simulink model "complementaryVsKalmanAndroidAHRS"  (R2019b)
settings: Solver=FixedStepAuto  StartTime=0.0  StopTime=40  RelTol=1e-3
InitFcn:
  | Ts=0.004
undefined symbols (not defined in the file): DiscIntNeverNeededParam
libraries: androiduilib x13, simulink_extras x11, dspstat3 x3, androidsensorlib x3
PreSaveFcn:
  | set_param(gcs, 'Location',[35 56 895 605])
settings Model: SimulationMode=external  ExtModeTrigDuration=100  Creator=The MathWorks, Inc.  LastModifiedBy=Alireza
settings DataIOCC: LimitDataPoints=on  SaveFormat=Array  ReturnWorkspaceOutputs=off
settings OptimizationCC: LifeSpan=1  MaxStackSize=64
settings DebuggingCC: UnderspecifiedInitializationDetection=Classic  MergeDetectMultiDrivingBlocksExec=none  ParameterPrecisionLossMsg=none  AllowSymbolicDim=off  SFUnexpectedBacktrackingDiag=warning  SFNoUnconditionalDefaultTransitionDiag=warning  SFExecutionAtInitializationDiag=none  ArithmeticOperatorsInVariantConditions=warning
settings HardwareCC: ProdBitPerPointer=32  ProdBitPerSizeT=32  ProdBitPerPtrDiffT=32  ProdLargestAtomicInteger=Long  ProdLargestAtomicFloat=Double  ProdWordSize=32  ProdHWDeviceType=ARM Compatible->ARM Cortex  TargetLargestAtomicInteger=Long  TargetLargestAtomicFloat=Double  TargetEndianess=LittleEndian  TargetHWDeviceType=ARM Compatible->ARM Cortex
settings ModelReferenceCC: PropagateSignalLabelsOutOfModel=off
settings SFSimCC: SimUseLocalCustomCode=off  CustomCodeUndefinedFunction=UseInterfaceOnly
settings RTWCC: SystemTargetFile=ert.tlc  HardwareBoard=Android Device  TLCOptions="-aInlineSetEventsForThisBaseRateFcn=TLC_FALSE -aSuppressMultiTaskScheduler=TLC_FALSE  -aRateBasedStepFcn=0"  TemplateMakefile=ert_default_tmf  GenerateReport=on  RTWVerbose=off  RTWUseLocalCustomCode=off  Toolchain=Android SDK/NDK Tools  LaunchReport=on
settings CodeAppCC: ForceParamTrailComments=on  OperatorAnnotations=on  MangleLength=10  StateflowObjectComments=on  MATLABSourceComments=on
settings ERTTargetCC: MultiwordLength=2048  ERTCustomFileBanners=off  SupportContinuousTime=on  SupportNonInlinedSFcns=on  RemoveResetFunc=off  SupportVariableSizeSignals=on  ModelStepFunctionPrototypeControlCompliant=off
settings ConfigComp: CovMetricSettings=dw  CovHtmlReporting=on  CovSaveCumulativeToWorkspaceVar=on  CovSaveSingleToWorkspaceVar=on  CovExternalEMLEnable=off  CovSFcnEnable=off

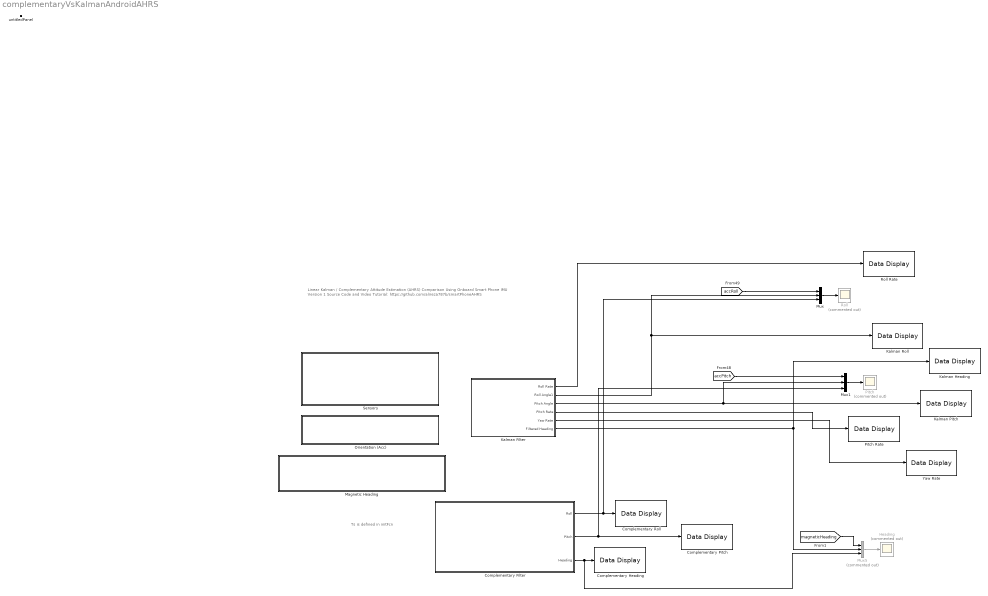
== system complementaryVsKalmanAndroidAHRS ==
  note: Ts is defined in initFcn
  note: Linear Kalman / Complementary Attitude Estimation (AHRS) Comparison
      | Using Onboard Smart Phone IMU Version 1
      | Source Code and Video Tutorial:
      | https://github.com/alireza787b/smartPhoneAHRS
  Complementary Filter : Subsystem
  Complementary Heading : androiduilib/Data Display  DataDisplayId=complementaryVsKalmanAndroidAHRS/Complementary_Heading  Format=Float  Precision=6  SimulateUsing=Code generation  blockPlatform=Android
      settings: SourceProductBaseCode=ANDROID
  Complementary Pitch : androiduilib/Data Display  DataDisplayId=complementaryVsKalmanAndroidAHRS/Complementary_Pitch  Format=Float  Precision=6  SimulateUsing=Code generation  blockPlatform=Android
      settings: SourceProductBaseCode=ANDROID
  Complementary Roll : androiduilib/Data Display  DataDisplayId=complementaryVsKalmanAndroidAHRS/Complementary_Roll  Format=Float  Precision=6  SimulateUsing=Code generation  blockPlatform=Android
      settings: SourceProductBaseCode=ANDROID
  Heading : Scope  Commented=on
  Kalman Filter : Subsystem
  "Kalman Heading " : androiduilib/Data Display  DataDisplayId=complementaryVsKalmanAndroidAHRS/Kalman_Heading_  Format=Float  Precision=6  SimulateUsing=Code generation  blockPlatform=Android
      settings: SourceProductBaseCode=ANDROID
  "Kalman Pitch " : androiduilib/Data Display  DataDisplayId=complementaryVsKalmanAndroidAHRS/Kalman_Pitch_  Format=Float  Precision=6  SimulateUsing=Code generation  blockPlatform=Android
      settings: SourceProductBaseCode=ANDROID
  Kalman Roll : androiduilib/Data Display  DataDisplayId=complementaryVsKalmanAndroidAHRS/Kalman_Roll  Format=Float  Precision=6  SimulateUsing=Code generation  blockPlatform=Android
      settings: SourceProductBaseCode=ANDROID
  Magnetic Heading : Subsystem
  Mux : Mux  Inputs=3
  Mux1 : Mux  Inputs=3
  Mux5 : Mux  Commented=on  Inputs=3
  Orientation (Acc) : Subsystem
  Pitch : Scope  Commented=on
  Pitch Rate : androiduilib/Data Display  DataDisplayId=complementaryVsKalmanAndroidAHRS/Pitch_Rate  Format=Float  Precision=6  SimulateUsing=Code generation  blockPlatform=Android
      settings: SourceProductBaseCode=ANDROID
  Roll : Scope  Commented=on
  Roll Rate : androiduilib/Data Display  DataDisplayId=complementaryVsKalmanAndroidAHRS/Roll_Rate  Format=Float  Precision=6  SimulateUsing=Code generation  blockPlatform=Android
      settings: SourceProductBaseCode=ANDROID
  Sensors : Subsystem
  Yaw Rate : androiduilib/Data Display  DataDisplayId=complementaryVsKalmanAndroidAHRS/Yaw_Rate  Format=Float  Precision=6  SimulateUsing=Code generation  blockPlatform=Android
      settings: SourceProductBaseCode=ANDROID
  untitledPanel : Subsystem  Tag=HiddenForWebPanel  IsWebBlockPanel=on
  wires:
  Mux/1 -> Roll/1
  Mux1/1 -> Pitch/1
  Mux5/1 -> Heading/1
  [accPitch] -> Mux1/1
  [accRoll] -> Mux/1
  Complementary Filter/1(Roll) -> Mux/3, Complementary Roll/1
  Complementary Filter/2("Pitch ") -> Complementary Pitch/1, Mux1/3
  Complementary Filter/3(Heading) -> Mux5/3, Complementary Heading/1
  Kalman Filter/2(Roll Angle1) -> Mux/2, Kalman Roll/1
  Kalman Filter/3(Pitch Angle) -> "Kalman Pitch "/1, Mux1/2
  Kalman Filter/6(Filtered Heading) -> Mux5/2, "Kalman Heading "/1
  Kalman Filter/1(Roll Rate) -> Roll Rate/1
  Kalman Filter/4(Pitch Rate) -> Pitch Rate/1
  Kalman Filter/5(Yaw Rate) -> Yaw Rate/1
  [magneticHeading] -> Mux5/1

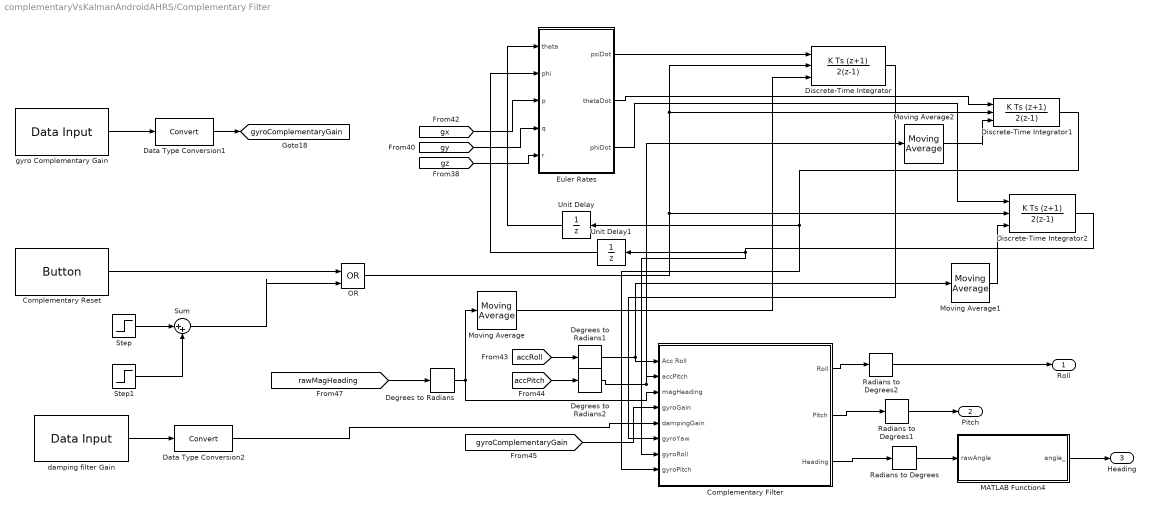
== system complementaryVsKalmanAndroidAHRS/Complementary Filter ==
  Complementary Filter : Subsystem
  Complementary Reset : androiduilib/Button  ButtonState=Not pressed  ButtonId=complementaryVsKalmanAndroidAHRS/Complementary_Filter/Complementary_Reset  State=off  SampleTime=0.1  BlockPlatform=Android
      settings: SourceProductBaseCode=ANDROID
  Data Type Conversion1 : DataTypeConversion
  Data Type Conversion2 : DataTypeConversion
  Degrees to Radians : simulink_extras/Transformations/Degrees to Radians
  Degrees to Radians1 : simulink_extras/Transformations/Degrees to Radians
  Degrees to Radians2 : simulink_extras/Transformations/Degrees to Radians
  Discrete-Time Integrator : DiscreteIntegrator  IntegratorMethod=Integration: Trapezoidal  ExternalReset=either  InitialConditionSource=external  SampleTime=-1  ICPrevOutput=DiscIntNeverNeededParam  ICPrevScaledInput=DiscIntNeverNeededParam
  Discrete-Time Integrator1 : DiscreteIntegrator  IntegratorMethod=Integration: Trapezoidal  ExternalReset=either  InitialConditionSource=external  SampleTime=-1  ICPrevOutput=DiscIntNeverNeededParam  ICPrevScaledInput=DiscIntNeverNeededParam
  Discrete-Time Integrator2 : DiscreteIntegrator  IntegratorMethod=Integration: Trapezoidal  ExternalReset=falling  InitialConditionSource=external  SampleTime=-1  ICPrevOutput=DiscIntNeverNeededParam  ICPrevScaledInput=DiscIntNeverNeededParam
  Euler Rates : Subsystem
  MATLAB Function4 : MATLAB Function  TreatAsAtomicUnit=on
  Moving Average : dspstat3/Moving Average  Method=Sliding window  ForgettingFactorPort=off  SpecifyWindowLength=on  WindowLength=4  ForgettingFactor=0.9  SimulateUsing=Code generation
  Moving Average1 : dspstat3/Moving Average  Method=Sliding window  ForgettingFactorPort=off  SpecifyWindowLength=on  WindowLength=4  ForgettingFactor=0.9  SimulateUsing=Code generation
  Moving Average2 : dspstat3/Moving Average  Method=Sliding window  ForgettingFactorPort=off  SpecifyWindowLength=on  WindowLength=4  ForgettingFactor=0.9  SimulateUsing=Code generation
  OR : Logic  Operator=OR  IconShape=distinctive  AllPortsSameDT=off  OutDataTypeStr=boolean
  Radians to Degrees : simulink_extras/Transformations/Radians to Degrees
  Radians to Degrees1 : simulink_extras/Transformations/Radians to Degrees
  Radians to Degrees2 : simulink_extras/Transformations/Radians to Degrees
  Step : Step  SampleTime=0
  Step1 : Step  Time=2  After=-1  SampleTime=0
  Sum : Sum  Inputs=|++
  Unit Delay : UnitDelay  SampleTime=-1  HasFrameUpgradeWarning=on
  Unit Delay1 : UnitDelay  SampleTime=-1  HasFrameUpgradeWarning=on
  damping filter Gain : androiduilib/Data Input  isCharVector=off  Value=0.9  CharVector=Hello World  OutputDataType=double  maxCharVectorSize=100  DataInputId=complementaryVsKalmanAndroidAHRS/Complementary_Filter/damping_filter_Gain  SampleTime=0.1
      settings: SourceProductBaseCode=ANDROID
  gyro Complementary Gain : androiduilib/Data Input  isCharVector=off  Value=0.78  CharVector=Hello World  OutputDataType=double  maxCharVectorSize=100  DataInputId=complementaryVsKalmanAndroidAHRS/Complementary_Filter/gyro_Complementary_Gain  SampleTime=0.1
      settings: SourceProductBaseCode=ANDROID
  Roll : Outport
  "Pitch " : Outport  Port=2
  Heading : Outport  Port=3
  tag scope: gyroComplementaryGain=global
  wires:
  [gy] -> Euler Rates/4(q)
  Euler Rates/3(phiDot) -> Discrete-Time Integrator2/1
  gyro Complementary Gain/1 -> Data Type Conversion1/1
  Complementary Filter/3(Heading) -> Radians to Degrees/1
  Euler Rates/1(psiDot) -> Discrete-Time Integrator/1
  Discrete-Time Integrator/1 -> Complementary Filter/6(gyroYaw)
  Unit Delay/1 -> Euler Rates/1(theta)
  Complementary Filter/1(Roll) -> Radians to Degrees2/1
  Unit Delay1/1 -> Euler Rates/2(phi)
  Degrees to Radians/1 -> Moving Average/1, Complementary Filter/3(magHeading)
  Discrete-Time Integrator1/1 -> Unit Delay/1, Complementary Filter/8(gyroPitch)
  [accRoll] -> Degrees to Radians1/1
  [gyroComplementaryGain] -> Complementary Filter/4(gyroGain)
  Discrete-Time Integrator2/1 -> Unit Delay1/1, Complementary Filter/7(gyroRoll)
  [rawMagHeading] -> Degrees to Radians/1
  [gx] -> Euler Rates/3(p)
  Euler Rates/2(thetaDot) -> Discrete-Time Integrator1/1
  [gz] -> Euler Rates/5(r)
  [accPitch] -> Degrees to Radians2/1
  Complementary Filter/2(Pitch) -> Radians to Degrees1/1
  Radians to Degrees1/1 -> "Pitch "/1
  Radians to Degrees2/1 -> Roll/1
  Radians to Degrees/1 -> MATLAB Function4/1(rawAngle)
  OR/1 -> Discrete-Time Integrator/2, Discrete-Time Integrator1/2, Discrete-Time Integrator2/2
  Moving Average/1 -> Discrete-Time Integrator/3
  Moving Average1/1 -> Discrete-Time Integrator2/3
  Moving Average2/1 -> Discrete-Time Integrator1/3
  Degrees to Radians1/1 -> Moving Average1/1, Complementary Filter/1(Acc Roll)
  Degrees to Radians2/1 -> Moving Average2/1, Complementary Filter/2(accPitch)
  MATLAB Function4/1(angle_) -> Heading/1
  Data Type Conversion1/1 -> [gyroComplementaryGain]
  Complementary Reset/1 -> OR/1
  Step/1 -> Sum/1
  Step1/1 -> Sum/2
  Sum/1 -> OR/2
  damping filter Gain/1 -> Data Type Conversion2/1
  Data Type Conversion2/1 -> Complementary Filter/5(dampingGain)

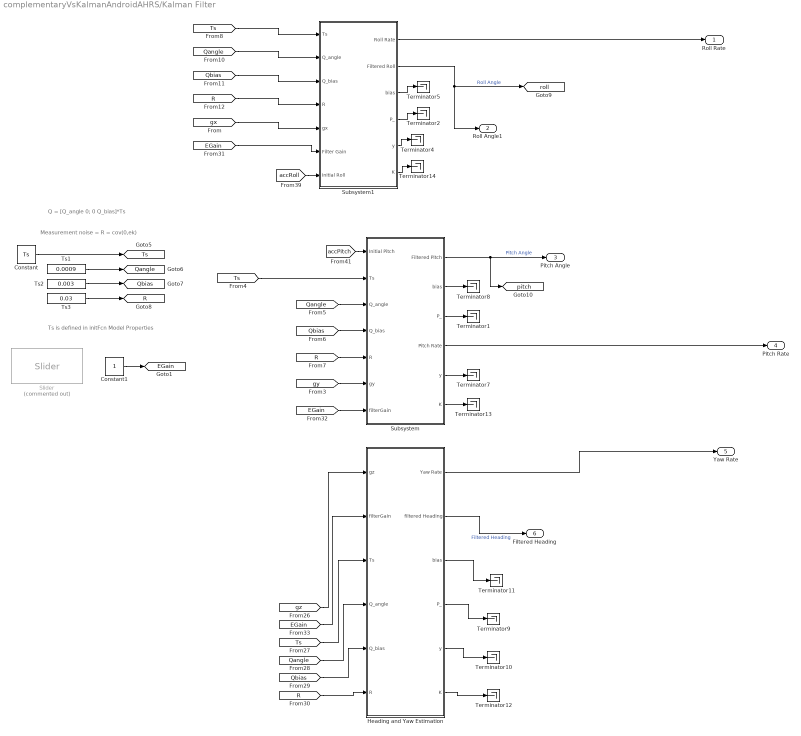
== system complementaryVsKalmanAndroidAHRS/Kalman Filter ==
  note: Q = [Q_angle 0; 0 Q_bias]*Ts
  note: Ts is defined in initFcn Model Properties
  note: Measurement noise = R = cov(0,ek)
  Constant : Constant  Value=Ts
  Constant1 : Constant
  Heading and Yaw Estimation : Subsystem
  Slider : androiduilib/Slider  Commented=on  Min=-2  Value=1  Max=2  Resolution=0.1  SliderId=kalmanAndroidAHRS/Kalman_Filter/Slider  SampleTime=0.1  BlockPlatform=Android
      settings: SourceProductBaseCode=ANDROID
  Subsystem : Subsystem
  Subsystem1 : Subsystem
  Terminator{1..2,4..5,7..14} (12 alike) : Terminator
  Ts1 : Constant  Value=0.0009
  Ts2 : Constant  Value=0.003
  Ts3 : Constant  Value=0.03
  Roll Rate : Outport
  Roll Angle1 : Outport  Port=2
  Pitch Angle : Outport  Port=3
  Pitch Rate : Outport  Port=4
  Yaw Rate : Outport  Port=5
  Filtered Heading : Outport  Port=6
  tag scope: EGain=global, Qangle=global, Qbias=global, R=global, Ts=global, pitch=global, roll=global
  wires:
  [R] -> Subsystem/5(R)
  Subsystem/5(y) -> Terminator7/1
  [R] -> Subsystem1/4(R)
  [Qbias] -> Subsystem/4(Q_bias)
  [Qangle] -> Subsystem1/2(Q_angle)
  Subsystem/2(bias) -> Terminator8/1
  [Qangle] -> Subsystem/3(Q_angle)
  [EGain] -> Heading and Yaw Estimation/2(filterGain)
  [EGain] -> Subsystem1/6(Filter Gain)
  [accPitch] -> Subsystem/1(Initial Pitch)
  Heading and Yaw Estimation/4(P_) -> Terminator9/1
  [Ts] -> Heading and Yaw Estimation/3(Ts)
  [R] -> Heading and Yaw Estimation/6(R)
  Subsystem/4(Pitch Rate) -> Pitch Rate/1
  [Qbias] -> Heading and Yaw Estimation/5(Q_bias)
  Subsystem1/6(K) -> Terminator14/1
  Heading and Yaw Estimation/1(Yaw Rate) -> Yaw Rate/1
  [accRoll] -> Subsystem1/7(Initial Roll)
  Subsystem/3(P_) -> Terminator1/1
  [gy] -> Subsystem/6(gy)
  Subsystem1/4(P_) -> Terminator2/1
  Heading and Yaw Estimation/2(filtered Heading) -> Filtered Heading/1  "Filtered Heading"
  [Ts] -> Subsystem/2(Ts)
  Subsystem/1(Filtered Pitch) -> Pitch Angle/1, [pitch]  "Pitch Angle"
  Heading and Yaw Estimation/3(bias) -> Terminator11/1
  [Qbias] -> Subsystem1/3(Q_bias)
  Heading and Yaw Estimation/6(K) -> Terminator12/1
  Subsystem1/5(y) -> Terminator4/1
  [gx] -> Subsystem1/5(gx)
  Subsystem1/3(bias) -> Terminator5/1
  Subsystem/6(K) -> Terminator13/1
  [Ts] -> Subsystem1/1(Ts)
  [Qangle] -> Heading and Yaw Estimation/4(Q_angle)
  Subsystem1/1(Roll Rate) -> Roll Rate/1
  [EGain] -> Subsystem/7(filterGain)
  Heading and Yaw Estimation/5(y) -> Terminator10/1
  Subsystem1/2(Filtered Roll) -> [roll], Roll Angle1/1  "Roll Angle"
  [gz] -> Heading and Yaw Estimation/1(gz)
  Ts2/1 -> [Qbias]
  Ts1/1 -> [Qangle]
  Ts3/1 -> [R]
  Constant/1 -> [Ts]
  Constant1/1 -> [EGain]

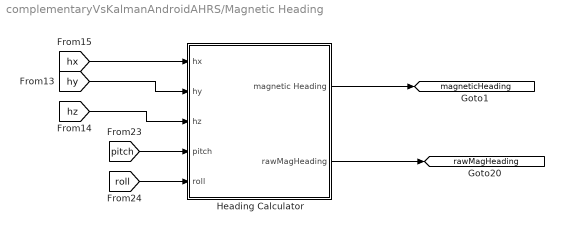
== system complementaryVsKalmanAndroidAHRS/Magnetic Heading ==
  Heading Calculator : Subsystem
  tag scope: magneticHeading=global, rawMagHeading=global
  wires:
  [hz] -> Heading Calculator/3(hz)
  [hy] -> Heading Calculator/2(hy)
  [hx] -> Heading Calculator/1(hx)
  [pitch] -> Heading Calculator/4(pitch)
  [roll] -> Heading Calculator/5(roll)
  Heading Calculator/2(rawMagHeading) -> [rawMagHeading]
  Heading Calculator/1(magnetic Heading) -> [magneticHeading]

== system complementaryVsKalmanAndroidAHRS/Orientation (Acc) ==
  Initial Angles by Accelerometer : Subsystem
  tag scope: accPitch=global, accRoll=global
  wires:
  [ax] -> Initial Angles by Accelerometer/1(X_value_of_Acc)
  Initial Angles by Accelerometer/2(Initial Pitch) -> [accPitch]
  [ay] -> Initial Angles by Accelerometer/2(Y_value_of_Acc)
  [az] -> Initial Angles by Accelerometer/3(Z_value_of_Acc)
  Initial Angles by Accelerometer/1(Initial Roll) -> [accRoll]

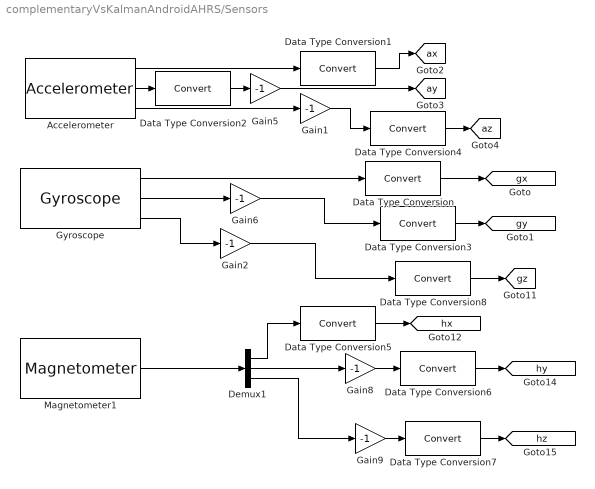
== system complementaryVsKalmanAndroidAHRS/Sensors ==
  Accelerometer : androidsensorlib/Accelerometer  OutputVector=off  SampleTime=Ts  BlockPlatform=Android
      settings: SourceProductBaseCode=ANDROID
  Data Type Conversion{,1..8} (9 alike) : DataTypeConversion
  Demux1 : Demux  Outputs=3
  Gain{1..2,5..6,8..9} (6 alike) : Gain  Gain=-1
  Gyroscope : androidsensorlib/Gyroscope  OutputVector=off  SampleTime=Ts  BlockPlatform=Android
      settings: SourceProductBaseCode=ANDROID
  Magnetometer1 : androidsensorlib/Magnetometer  SampleTime=0.01  SimulateUsing=Code generation
      settings: SourceProductBaseCode=ANDROID
  tag scope: ax=global, ay=global, az=global, gx=global, gy=global, gz=global, hx=global, hy=global, hz=global
  wires:
  Demux1/1 -> Data Type Conversion5/1
  Gain8/1 -> Data Type Conversion6/1
  Data Type Conversion6/1 -> [hy]
  Accelerometer/2 -> Data Type Conversion2/1
  Demux1/3 -> Gain9/1
  Data Type Conversion5/1 -> [hx]
  Gain1/1 -> Data Type Conversion4/1
  Accelerometer/3 -> Gain1/1
  Gyroscope/2 -> Gain6/1
  Data Type Conversion7/1 -> [hz]
  Gain2/1 -> Data Type Conversion8/1
  Data Type Conversion4/1 -> [az]
  Gyroscope/1 -> Data Type Conversion/1
  Data Type Conversion3/1 -> [gy]
  Gain9/1 -> Data Type Conversion7/1
  Gain5/1 -> [ay]
  Data Type Conversion/1 -> [gx]
  Magnetometer1/1 -> Demux1/1
  Gain6/1 -> Data Type Conversion3/1
  Accelerometer/1 -> Data Type Conversion1/1
  Gyroscope/3 -> Gain2/1
  Demux1/2 -> Gain8/1
  Data Type Conversion8/1 -> [gz]
  Data Type Conversion2/1 -> Gain5/1
  Data Type Conversion1/1 -> [ax]

== system complementaryVsKalmanAndroidAHRS/untitledPanel ==
  Half Gauge : SemiCircularGaugeBlock  Tag=HiddenForWebPanel  PanelInfo="{\"panelId\":\"panelId-765474a9-9c5b-495a-8d41-f66c7c8f1f34\",\"type\":\"panelChild\",\"version\":\"2019b\",\"zIndex\":1500004}"  ScaleMin=-90  ScaleMax=+90
  Half Gauge1 : SemiCircularGaugeBlock  Tag=HiddenForWebPanel  PanelInfo="{\"panelId\":\"panelId-765474a9-9c5b-495a-8d41-f66c7c8f1f34\",\"type\":\"panelChild\",\"version\":\"2019b\",\"zIndex\":1500001}"  ScaleMin=-90  ScaleMax=+90
  Half Gauge2 : SemiCircularGaugeBlock  Tag=HiddenForWebPanel  PanelInfo="{\"panelId\":\"panelId-765474a9-9c5b-495a-8d41-f66c7c8f1f34\",\"type\":\"panelChild\",\"version\":\"2019b\",\"zIndex\":1500002}"  ScaleMax=360
  panelInfo : PanelWebBlock  Tag=HiddenForWebPanel  PanelInfo="{\"compacted\":true,\"height\":441,\"labels\":{\"label8769572146\":{\"left\":\"231\",\"settings\":{\"backgroundColor\":\"rgba(0, 0, 0, 0)\",\"bold\":false,\"font\":\"Arial\",\"fontColor\":\"black\",\"fontSize\":1.48,\"italicized\":false,\"underlined\":false},\"text\":\"\\u001B\\u001B\",\"top\":\"319\"}},\"left\":1290,\"panelId\":\"panelId-765474a9-9c5b-495a-8d41-f66c7c8f1f34\",\"top\":463,\"type\":\"panel\",\"version\":\"2019b\",\"visible\":true,\"width\":432,\"zIndex\":1500001}"  PanelSnapshot=<binary blob, 68872 chars, not shown>

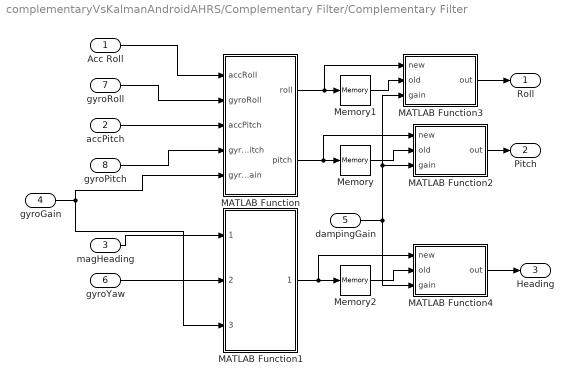
== system complementaryVsKalmanAndroidAHRS/Complementary Filter/Complementary Filter ==
  Acc Roll : Inport
  accPitch : Inport  Port=2
  magHeading : Inport  Port=3
  gyroGain : Inport  Port=4
  dampingGain : Inport  Port=5
  gyroYaw : Inport  Port=6
  gyroRoll : Inport  Port=7
  gyroPitch : Inport  Port=8
  MATLAB Function : MATLAB Function  TreatAsAtomicUnit=on
  MATLAB Function1 : MATLAB Function  TreatAsAtomicUnit=on
  MATLAB Function2 : MATLAB Function  TreatAsAtomicUnit=on
  MATLAB Function3 : MATLAB Function  TreatAsAtomicUnit=on
  MATLAB Function4 : MATLAB Function  TreatAsAtomicUnit=on
  Memory : Memory
  Memory1 : Memory
  Memory2 : Memory
  Roll : Outport
  Pitch : Outport  Port=2
  Heading : Outport  Port=3
  wires:
  MATLAB Function/2(pitch) -> MATLAB Function2/1(new), Memory/1
  gyroPitch/1 -> MATLAB Function/4(gyroPitch)
  accPitch/1 -> MATLAB Function/3(accPitch)
  gyroRoll/1 -> MATLAB Function/2(gyroRoll)
  Acc Roll/1 -> MATLAB Function/1(accRoll)
  gyroYaw/1 -> MATLAB Function1/2(gyroYaw)
  magHeading/1 -> MATLAB Function1/1(magHeading)
  MATLAB Function1/1(heading) -> MATLAB Function4/1(new), Memory2/1
  MATLAB Function/1(roll) -> MATLAB Function3/1(new), Memory1/1
  Memory/1 -> MATLAB Function2/2(old)
  MATLAB Function2/1(out) -> Pitch/1
  MATLAB Function3/1(out) -> Roll/1
  Memory1/1 -> MATLAB Function3/2(old)
  Memory2/1 -> MATLAB Function4/2(old)
  MATLAB Function4/1(out) -> Heading/1
  gyroGain/1 -> MATLAB Function1/3(gyroGainHeading), MATLAB Function/5(gyroGain)
  dampingGain/1 -> MATLAB Function3/3(gain), MATLAB Function2/3(gain), MATLAB Function4/3(gain)

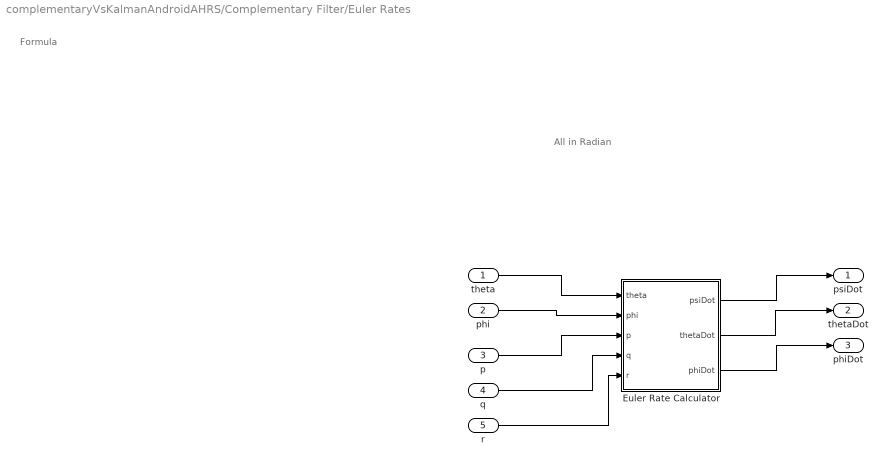
== system complementaryVsKalmanAndroidAHRS/Complementary Filter/Euler Rates ==
  note: All in Radian
  note: Formula
  theta : Inport
  phi : Inport  Port=2
  p : Inport  Port=3
  q : Inport  Port=4
  r : Inport  Port=5
  Euler Rate Calculator : MATLAB Function  TreatAsAtomicUnit=on
  psiDot : Outport
  thetaDot : Outport  Port=2
  phiDot : Outport  Port=3
  wires:
  phi/1 -> Euler Rate Calculator/2(phi)
  theta/1 -> Euler Rate Calculator/1(theta)
  p/1 -> Euler Rate Calculator/3(p)
  q/1 -> Euler Rate Calculator/4(q)
  r/1 -> Euler Rate Calculator/5(r)
  Euler Rate Calculator/1(psiDot) -> psiDot/1
  Euler Rate Calculator/2(thetaDot) -> thetaDot/1
  Euler Rate Calculator/3(phiDot) -> phiDot/1

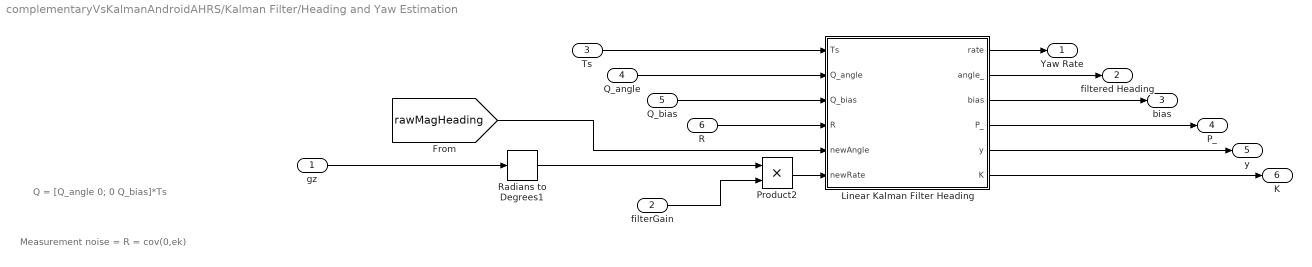
== system complementaryVsKalmanAndroidAHRS/Kalman Filter/Heading and Yaw Estimation ==
  note: Measurement noise = R = cov(0,ek)
  note: Q = [Q_angle 0; 0 Q_bias]*Ts
  gz : Inport
  filterGain : Inport  Port=2
  Ts : Inport  Port=3
  Q_angle : Inport  Port=4
  Q_bias : Inport  Port=5
  R : Inport  Port=6
  Linear Kalman Filter Heading : MATLAB Function  TreatAsAtomicUnit=on
  Product2 : Product
  Radians to Degrees1 : simulink_extras/Transformations/Radians to Degrees
  Yaw Rate : Outport
  filtered Heading : Outport  Port=2
  bias : Outport  Port=3
  P_ : Outport  Port=4
  y : Outport  Port=5
  K : Outport  Port=6
  wires:
  Linear Kalman Filter Heading/2(angle_) -> filtered Heading/1
  Product2/1 -> Linear Kalman Filter Heading/6(newRate)
  Linear Kalman Filter Heading/6(K) -> K/1
  Q_angle/1 -> Linear Kalman Filter Heading/2(Q_angle)
  gz/1 -> Radians to Degrees1/1
  Ts/1 -> Linear Kalman Filter Heading/1(Ts)
  R/1 -> Linear Kalman Filter Heading/4(R)
  Linear Kalman Filter Heading/3(bias) -> bias/1
  Linear Kalman Filter Heading/1(rate) -> Yaw Rate/1
  filterGain/1 -> Product2/2
  Q_bias/1 -> Linear Kalman Filter Heading/3(Q_bias)
  Linear Kalman Filter Heading/5(y) -> y/1
  Linear Kalman Filter Heading/4(P_) -> P_/1
  Radians to Degrees1/1 -> Product2/1
  [rawMagHeading] -> Linear Kalman Filter Heading/5(newAngle)

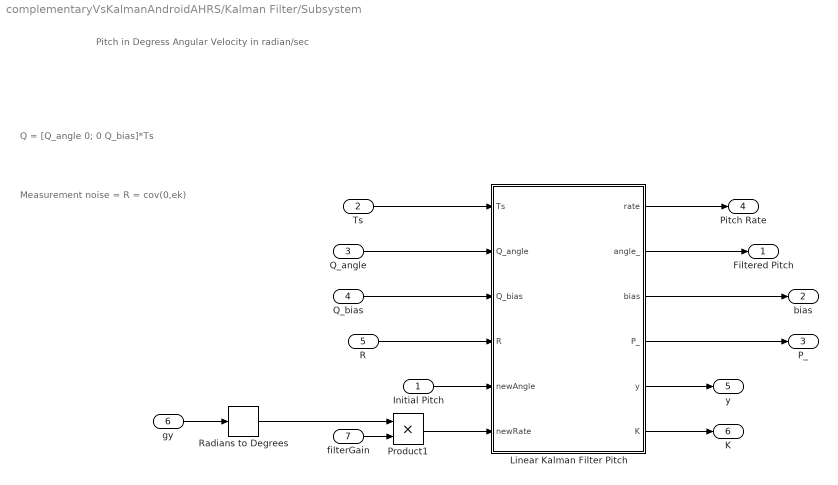
== system complementaryVsKalmanAndroidAHRS/Kalman Filter/Subsystem ==
  note: Pitch in Degress
      | Angular Velocity in radian/sec
  note: Measurement noise = R = cov(0,ek)
  note: Q = [Q_angle 0; 0 Q_bias]*Ts
  Initial Pitch : Inport
  Ts : Inport  Port=2
  Q_angle : Inport  Port=3
  Q_bias : Inport  Port=4
  R : Inport  Port=5
  gy : Inport  Port=6
  filterGain : Inport  Port=7
  Linear Kalman Filter Pitch : MATLAB Function  TreatAsAtomicUnit=on
  Product1 : Product
  Radians to Degrees : simulink_extras/Transformations/Radians to Degrees
  Filtered Pitch : Outport
  bias : Outport  Port=2
  P_ : Outport  Port=3
  Pitch Rate : Outport  Port=4
  y : Outport  Port=5
  K : Outport  Port=6
  wires:
  Linear Kalman Filter Pitch/3(bias) -> bias/1
  Linear Kalman Filter Pitch/1(rate) -> Pitch Rate/1
  Product1/1 -> Linear Kalman Filter Pitch/6(newRate)
  filterGain/1 -> Product1/2
  gy/1 -> Radians to Degrees/1
  Linear Kalman Filter Pitch/5(y) -> y/1
  Linear Kalman Filter Pitch/4(P_) -> P_/1
  Ts/1 -> Linear Kalman Filter Pitch/1(Ts)
  Q_bias/1 -> Linear Kalman Filter Pitch/3(Q_bias)
  Q_angle/1 -> Linear Kalman Filter Pitch/2(Q_angle)
  Linear Kalman Filter Pitch/2(angle_) -> Filtered Pitch/1
  Linear Kalman Filter Pitch/6(K) -> K/1
  R/1 -> Linear Kalman Filter Pitch/4(R)
  Initial Pitch/1 -> Linear Kalman Filter Pitch/5(newAngle)
  Radians to Degrees/1 -> Product1/1

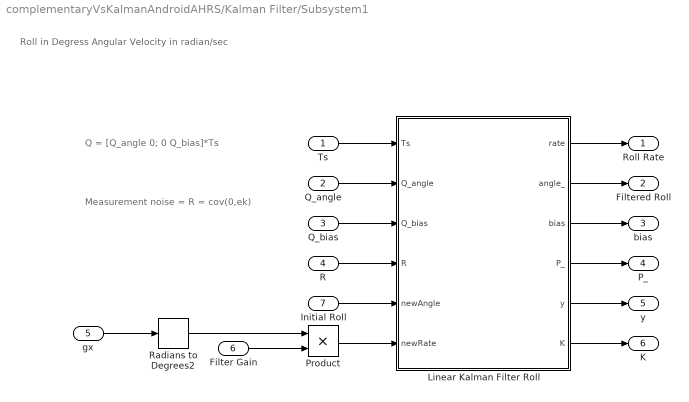
== system complementaryVsKalmanAndroidAHRS/Kalman Filter/Subsystem1 ==
  note: Measurement noise = R = cov(0,ek)
  note: Q = [Q_angle 0; 0 Q_bias]*Ts
  note: Roll in Degress
      | Angular Velocity in radian/sec
  Ts : Inport
  Q_angle : Inport  Port=2
  Q_bias : Inport  Port=3
  R : Inport  Port=4
  gx : Inport  Port=5
  Filter Gain : Inport  Port=6
  Initial Roll : Inport  Port=7
  Linear Kalman Filter Roll : MATLAB Function  TreatAsAtomicUnit=on
  Product : Product
  Radians to Degrees2 : simulink_extras/Transformations/Radians to Degrees
  Roll Rate : Outport
  Filtered Roll : Outport  Port=2
  bias : Outport  Port=3
  P_ : Outport  Port=4
  y : Outport  Port=5
  K : Outport  Port=6
  wires:
  Linear Kalman Filter Roll/4(P_) -> P_/1
  Linear Kalman Filter Roll/1(rate) -> Roll Rate/1
  Filter Gain/1 -> Product/2
  Linear Kalman Filter Roll/3(bias) -> bias/1
  Linear Kalman Filter Roll/5(y) -> y/1
  Product/1 -> Linear Kalman Filter Roll/6(newRate)
  Initial Roll/1 -> Linear Kalman Filter Roll/5(newAngle)
  R/1 -> Linear Kalman Filter Roll/4(R)
  Q_bias/1 -> Linear Kalman Filter Roll/3(Q_bias)
  Q_angle/1 -> Linear Kalman Filter Roll/2(Q_angle)
  Linear Kalman Filter Roll/6(K) -> K/1
  gx/1 -> Radians to Degrees2/1
  Linear Kalman Filter Roll/2(angle_) -> Filtered Roll/1
  Ts/1 -> Linear Kalman Filter Roll/1(Ts)
  Radians to Degrees2/1 -> Product/1

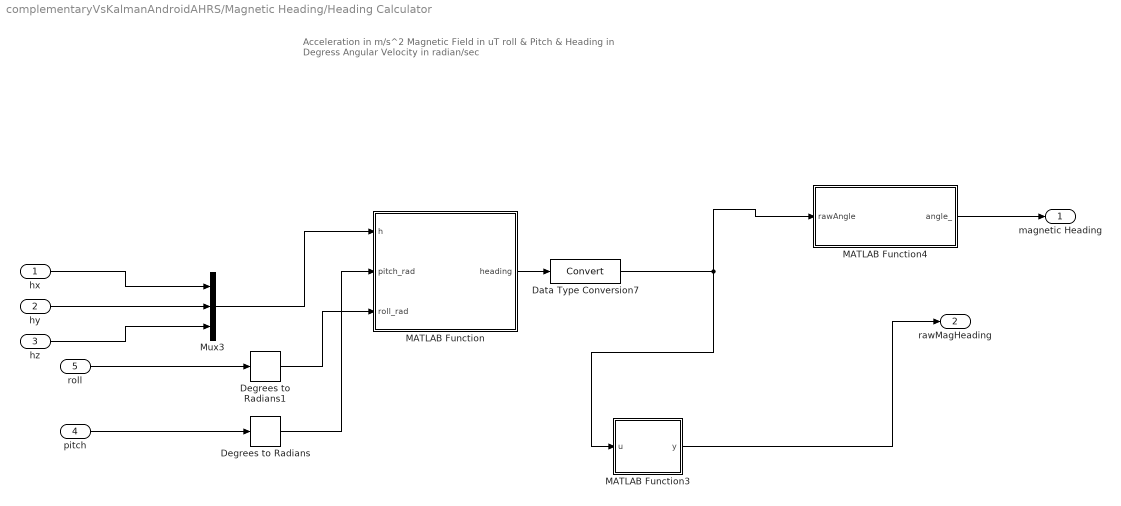
== system complementaryVsKalmanAndroidAHRS/Magnetic Heading/Heading Calculator ==
  note: Acceleration in m/s^2
      | Magnetic Field in uT
      | roll & Pitch & Heading in Degress
      | Angular Velocity in radian/sec
  hx : Inport
  hy : Inport  Port=2
  hz : Inport  Port=3
  pitch : Inport  Port=4
  roll : Inport  Port=5
  Data Type Conversion7 : DataTypeConversion
  Degrees to Radians : simulink_extras/Transformations/Degrees to Radians
  Degrees to Radians1 : simulink_extras/Transformations/Degrees to Radians
  MATLAB Function : MATLAB Function  TreatAsAtomicUnit=on
  MATLAB Function3 : MATLAB Function  TreatAsAtomicUnit=on
  MATLAB Function4 : MATLAB Function  TreatAsAtomicUnit=on
  Mux3 : Mux  Inputs=3
  magnetic Heading : Outport
  rawMagHeading : Outport  Port=2
  wires:
  hy/1 -> Mux3/2
  MATLAB Function3/1(y) -> rawMagHeading/1
  MATLAB Function/1(heading) -> Data Type Conversion7/1
  roll/1 -> Degrees to Radians1/1
  Data Type Conversion7/1 -> MATLAB Function3/1(u), MATLAB Function4/1(rawAngle)
  MATLAB Function4/1(angle_) -> magnetic Heading/1
  Mux3/1 -> MATLAB Function/1(h)
  Degrees to Radians/1 -> MATLAB Function/2(pitch_rad)
  Degrees to Radians1/1 -> MATLAB Function/3(roll_rad)
  hz/1 -> Mux3/3
  pitch/1 -> Degrees to Radians/1
  hx/1 -> Mux3/1

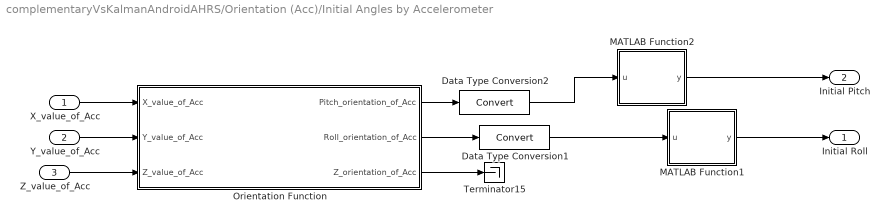
== system complementaryVsKalmanAndroidAHRS/Orientation (Acc)/Initial Angles by Accelerometer ==
  X_value_of_Acc : Inport
  Y_value_of_Acc : Inport  Port=2
  Z_value_of_Acc : Inport  Port=3
  Data Type Conversion1 : DataTypeConversion
  Data Type Conversion2 : DataTypeConversion
  MATLAB Function1 : MATLAB Function  TreatAsAtomicUnit=on
  MATLAB Function2 : MATLAB Function  TreatAsAtomicUnit=on
  Orientation Function : MATLAB Function  TreatAsAtomicUnit=on
  Terminator15 : Terminator
  Initial Roll : Outport
  Initial Pitch : Outport  Port=2
  wires:
  Orientation Function/2(Roll_orientation_of_Acc) -> Data Type Conversion1/1
  Data Type Conversion1/1 -> MATLAB Function1/1(u)
  X_value_of_Acc/1 -> Orientation Function/1(X_value_of_Acc)
  Y_value_of_Acc/1 -> Orientation Function/2(Y_value_of_Acc)
  Orientation Function/1(Pitch_orientation_of_Acc) -> Data Type Conversion2/1
  MATLAB Function2/1(y) -> Initial Pitch/1
  Data Type Conversion2/1 -> MATLAB Function2/1(u)
  Orientation Function/3(Z_orientation_of_Acc) -> Terminator15/1
  Z_value_of_Acc/1 -> Orientation Function/3(Z_value_of_Acc)
  MATLAB Function1/1(y) -> Initial Roll/1

== matlab function complementaryVsKalmanAndroidAHRS/Kalman Filter/Subsystem/Linear Kalman Filter Pitch ==
  data: Ts input; Q_angle input; Q_bias input; R input; newAngle input; rate output; newRate input; angle_ output; bias output; P_ output; y output; K output
% Algorithm -- implimentation of Linear-Kalman filter for a 6-DOF IMU using
% a single axis for testing. A single axis consisting of both anaccelerometer
% input and gyroscope input from IMU.
% Author: RM van Rensburg
% for IMU testing purposes
% Date: 26-04-2015
% Version: 1.0,tested on Matlab R2015a

function [rate,angle_,bias,P_,y,K] = Kalmanf(Ts,...
                                             Q_angle,Q_bias,R,...
                                             newAngle,...
                                             newRate)
                      
% Process noise covariance matrix  
Q = [Q_angle 0;0 Q_bias]*Ts;
A = [1  -Ts;0  1];
C = [1 0];
bias = 0.0;

rate = newRate - bias;

persistent angle;
if isempty(angle);angle = 0;
else angle = angle + (Ts * rate); 
end
angle_= angle;
                    
persistent P;
if isempty(P);P = [0 0 ; 0 0]; 
else P = A*P*A' + Q;
end
P_=P;

S = C*P*C' + R; % Estimate error 
K = (P_*C')/S; % Kalman gain
y = newAngle - angle_; % Angle difference 
xk = angle_ + K*y;
angle_ = xk(1); % - is added by me
bias = xk(2);
angle = angle_;

% Update the error covariance 
I = [1 0;0 1];
P_ = (I - K*C)*P_;
% or
% Joseph form (more stable)
% P_ = (I - K*C)*P_*(I - K*C) + K*R*K';
P = P_;

return

end

== matlab function complementaryVsKalmanAndroidAHRS/Orientation (Acc)/Initial Angles by Accelerometer/MATLAB Function2 ==
  data: u input; y output
function y = fcn(u)

if(isnan(u))
y=0;
else
y=u;
end

== matlab function complementaryVsKalmanAndroidAHRS/Orientation (Acc)/Initial Angles by Accelerometer/Orientation Function ==
  data: X_value_of_Acc input; Pitch_orientation_of_Acc output; Roll_orientation_of_Acc output; Z_orientation_of_Acc output; Y_value_of_Acc input; Z_value_of_Acc input
% Computing orientation of tri-axial acclerometer data from IMU 
% Author: RM van Rensburg
% Date: 26-04-2015
% Version: 1.0,tested on Matlab R2015a

function [Pitch_orientation_of_Acc,...
          Roll_orientation_of_Acc,...
          Z_orientation_of_Acc]...
          = OrientationFcn(X_value_of_Acc,Y_value_of_Acc,Z_value_of_Acc)
     
      
% Using x and y from accelerometer (g-forces), calculate x and y angles
% Data directly obtained from IMU
% Using the following formulae
% Ax = arctan{X/sqrt(Y*Y + Z*Z)}
% Ay = arctan{Y/sqrt(X*X + Z*Z)}

% Computing the X*X, Y*Y, Z*Z
X2 = power(X_value_of_Acc,2);
Y2 = power(Y_value_of_Acc,2);
Z2 = power(Z_value_of_Acc,2);

% x-axis angle
result = sqrt(Y2 + Z2);
result = X_value_of_Acc / result;
x_angle_rad = atan(result);
Pitch_orientation_of_Acc = (x_angle_rad * 180) / pi;

% y-axis angle
result = sqrt(X2 + Z2);
result = Y_value_of_Acc / result;
y_angle_rad = atan(result);
Roll_orientation_of_Acc = -(y_angle_rad * 180) / pi;

% z-axis angle
result = sqrt(Y2 + X2);
result = Z_value_of_Acc / result;
z_angle_rad = atan(result);
Z_orientation_of_Acc = (z_angle_rad * 180) / pi;

end

== matlab function complementaryVsKalmanAndroidAHRS/Orientation (Acc)/Initial Angles by Accelerometer/MATLAB Function1 ==
  data: u input; y output
function y = fcn(u)

if(isnan(u))
y=0;
else
y=u;
end

== matlab function complementaryVsKalmanAndroidAHRS/Kalman Filter/Subsystem1/Linear Kalman Filter Roll ==
  data: Ts input; Q_angle input; Q_bias input; R input; newAngle input; rate output; newRate input; angle_ output; bias output; P_ output; y output; K output
% Algorithm -- implimentation of Linear-Kalman filter for a 6-DOF IMU using
% a single axis for testing. A single axis consisting of both anaccelerometer
% input and gyroscope input from IMU.
% Author: RM van Rensburg
% for IMU testing purposes
% Date: 26-04-2015
% Version: 1.0,tested on Matlab R2015a

function [rate,angle_,bias,P_,y,K] = Kalmanf(Ts,...
                                             Q_angle,Q_bias,R,...
                                             newAngle,...
                                             newRate)
                      
% Process noise covariance matrix  
Q = [Q_angle 0;0 Q_bias]*Ts;
A = [1  -Ts;0  1];
C = [1 0];
bias = 0.0;

rate = newRate - bias;

persistent angle;
if isempty(angle);angle = 0;
else angle = angle + (Ts * rate); 
end
angle_= angle;
                    
persistent P;
if isempty(P);P = [0 0 ; 0 0]; 
else P = A*P*A' + Q;
end
P_=P;

S = C*P*C' + R; % Estimate error 
K = (P_*C')/S; % Kalman gain
y = newAngle - angle_; % Angle difference 
xk = angle_ + K*y;
angle_ = xk(1);
bias = xk(2);
angle = angle_;

% Update the error covariance 
I = [1 0;0 1];
P_ = (I - K*C)*P_;
% or
% Joseph form (more stable)
% P_ = (I - K*C)*P_*(I - K*C) + K*R*K';
P = P_;

return

end

== matlab function complementaryVsKalmanAndroidAHRS/Kalman Filter/Heading and Yaw Estimation/Linear Kalman Filter Heading ==
  data: Ts input; Q_angle input; Q_bias input; R input; newAngle input; rate output; newRate input; angle_ output; bias output; P_ output; y output; K output
% Algorithm -- implimentation of Linear-Kalman filter for a 6-DOF IMU using
% a single axis for testing. A single axis consisting of both anaccelerometer
% input and gyroscope input from IMU.
% Author: RM van Rensburg
% for IMU testing purposes
% Date: 26-04-2015
% Version: 1.0,tested on Matlab R2015a

function [rate,angle_,bias,P_,y,K] = Kalmanf(Ts,...
                                             Q_angle,Q_bias,R,...
                                             newAngle,...
                                             newRate)
                      
% Process noise covariance matrix  
Q = [Q_angle 0;0 Q_bias]*Ts;
A = [1  -Ts;0  1];
C = [1 0];
bias = 0.0;

rate = newRate - bias;

persistent angle;
if isempty(angle);angle = 0;
else angle = angle + (Ts * rate); 
end
 
angle_= angle;


                    
persistent P;
if isempty(P);P = [0 0 ; 0 0]; 
else P = A*P*A' + Q;
end
P_=P;

S = C*P*C' + R; % Estimate error 
K = (P_*C')/S; % Kalman gain
y = newAngle - angle_; % Angle difference 
xk = angle_ + K*y;
angle_ = xk(1);

bias = xk(2);
angle = angle_;

% Update the error covariance 
I = [1 0;0 1];
P_ = (I - K*C)*P_;
% or
% Joseph form (more stable)
% P_ = (I - K*C)*P_*(I - K*C) + K*R*K';
P = P_;


    if angle_ > 360 
        angle_ = angle_ - 360;
    elseif angle_ < 0
       angle_ =  angle_ + 360;
    end

return

end

== matlab function complementaryVsKalmanAndroidAHRS/Complementary Filter/MATLAB Function4 ==
  data: rawAngle input; angle_ output
function angle_ = constrainerHeading(rawAngle)
angle_ = rawAngle;
    if rawAngle > 360 ;
        angle_ = rawAngle - 360;
    elseif angle_ < 0;
       angle_ =  rawAngle + 360;
    end
end

== matlab function complementaryVsKalmanAndroidAHRS/Complementary Filter/Euler Rates/Euler Rate Calculator ==
  data: theta input; psiDot output; phi input; p input; q input; r input; thetaDot output; phiDot output
function [psiDot,thetaDot,phiDot] = fcn(theta,phi,p,q,r)

psiDot =  sin(phi)/cos(theta)*q + cos(phi)/cos(theta)*r;
thetaDot = cos(phi)*q - sin(phi)*r;
phiDot = p + sin(phi)*tan(theta)*q + cos(phi)*tan(theta)*r;
end

== matlab function complementaryVsKalmanAndroidAHRS/Complementary Filter/Complementary Filter/MATLAB Function ==
  data: accRoll input; roll output; gyroRoll input; accPitch input; gyroPitch input; gyroGain input; pitch output
function [roll,pitch] = fcn(accRoll,gyroRoll,accPitch,gyroPitch,gyroGain)
roll = gyroGain * gyroRoll + (1-gyroGain)*accRoll;
pitch = gyroGain * gyroPitch + (1-gyroGain)*accPitch;

end

== matlab function complementaryVsKalmanAndroidAHRS/Complementary Filter/Complementary Filter/MATLAB Function1 ==
  data: magHeading input; heading output; gyroYaw input; gyroGainHeading input
function heading  = headingCalc(magHeading,gyroYaw,gyroGainHeading)
heading = gyroGainHeading * gyroYaw + (1-gyroGainHeading)*magHeading;
end

== matlab function complementaryVsKalmanAndroidAHRS/Complementary Filter/Complementary Filter/MATLAB Function2 ==
  data: new input; out output; old input; gain input
function out = damper(new,old,gain)
out = gain * old + (1-gain)*new;
end

== matlab function complementaryVsKalmanAndroidAHRS/Complementary Filter/Complementary Filter/MATLAB Function3 ==
  data: new input; out output; old input; gain input
function out = damper(new,old,gain)
out = gain * old + (1-gain)*new;
end

== matlab function complementaryVsKalmanAndroidAHRS/Complementary Filter/Complementary Filter/MATLAB Function4 ==
  data: new input; out output; old input; gain input
function out = damper(new,old,gain)
out = gain * old + (1-gain)*new;
end

== matlab function complementaryVsKalmanAndroidAHRS/Magnetic Heading/Heading Calculator/MATLAB Function ==
  data: heading output; h input; pitch_rad input; roll_rad input
function heading  = mag2Heading(h,pitch_rad,roll_rad)
 h = normalize(h,'norm');
   
    heading_rad = atan2(h(3) * sin(roll_rad) - h(2) * cos(roll_rad), h(1) * cos(pitch_rad) + h(2) * sin(pitch_rad) * sin(roll_rad) + h(3) * sin(pitch_rad) * cos(roll_rad));
    heading = rad2deg(heading_rad);

== matlab function complementaryVsKalmanAndroidAHRS/Magnetic Heading/Heading Calculator/MATLAB Function3 ==
  data: u input; y output
function y = fcn(u)

if(isnan(u))
y=0;
else
y=u;
end

== matlab function complementaryVsKalmanAndroidAHRS/Magnetic Heading/Heading Calculator/MATLAB Function4 ==
  data: rawAngle input; angle_ output
function angle_ = constrainerHeading(rawAngle)
angle_ = rawAngle;
    if rawAngle > 360 ;
        angle_ = rawAngle - 360;
    elseif angle_ < 0;
       angle_ =  rawAngle + 360;
    end
end
